simulink model "BPSK_Simulink"  (R2021a)
settings: Solver=VariableStepAuto  StartTime=0.0  StopTime=10.0  RelTol=1e-3
libraries: commdigbbndpm3 x2, commchan3 x1, commsink2 x1, commrandsrc3 x1
settings Model: Creator=DAN  LastModifiedBy=DAN

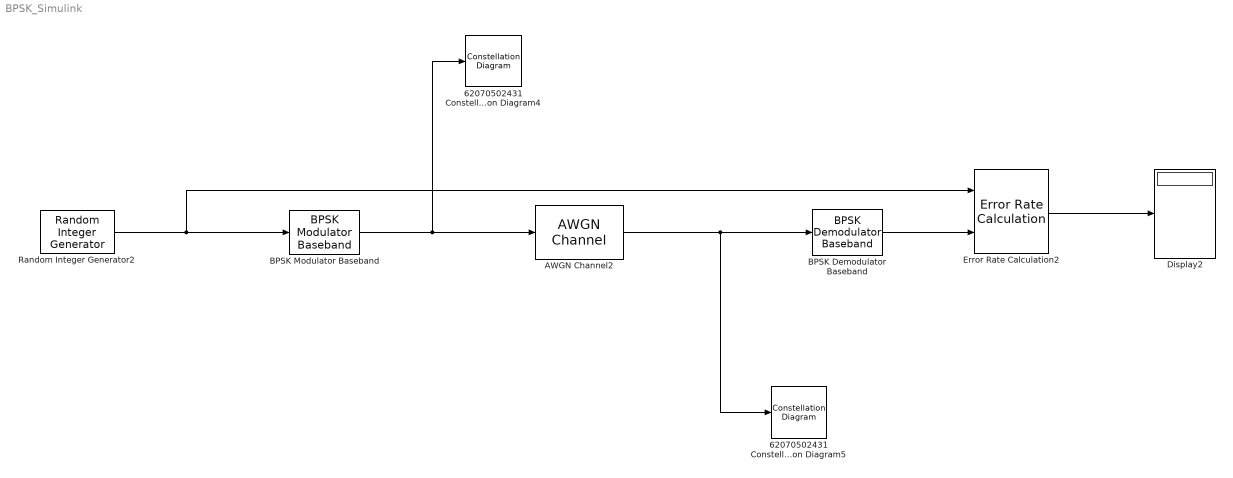
== system BPSK_Simulink ==
  62070502431 Constellation Diagram4 : ConstellationDiagram
  62070502431 Constellation Diagram5 : ConstellationDiagram
  AWGN Channel2 : commchan3/AWGN Channel  InputProcessing=Columns as channels (frame based)  seed=67  noiseMode="Signal to noise ratio  (Eb/No)"  EbNodB=3  EsNodB=10  SNRdB=10  bitsPerSym=1  Ps=1  Tsym=1e-6  variance=1
  BPSK Demodulator Baseband : commdigbbndpm3/BPSK Demodulator Baseband  DecType=Hard decision  VarSource=Dialog  Variance=1  Ph=0  outDtype=Inherit via internal rule  derotateFactorWordLen=16  derotateFactorDataTypeStr=Inherit: Same word length as input  derotateFactorLastDataTypeStr=Inherit: Same word length as input
  BPSK Modulator Baseband : commdigbbndpm3/BPSK Modulator Baseband  Ph=0  outDtype=double  outWordLen=16  outUDDataType=sfix(16)  outFracLenMode=Best precision  outFracLen=15  outDataTypeStr=double  outLastDataTypeStr=double
  Display2 : Display
  Error Rate Calculation2 : commsink2/Error Rate Calculation  N=0  st_delay=0  cp_mode=Entire frame  subframe=[]  PMode=Port  WsName=ErrorVec  RsMode2=off  stop=off  numErr=100  maxBits=1e6
  Random Integer Generator2 : commrandsrc3/Random Integer Generator  SetSize=2  SeedSource=Auto  Seed=0  SampleTime=1e-6  SamplesPerFrame=1024  OutputDataType=double  SimulateUsing=Interpreted execution
  wires:
  Random Integer Generator2/1 -> BPSK Modulator Baseband/1, Error Rate Calculation2/1
  AWGN Channel2/1 -> BPSK Demodulator Baseband/1, 62070502431 Constellation Diagram5/1
  BPSK Demodulator Baseband/1 -> Error Rate Calculation2/2
  Error Rate Calculation2/1 -> Display2/1
  BPSK Modulator Baseband/1 -> 62070502431 Constellation Diagram4/1, AWGN Channel2/1
